simulink model "model_2"  (R2023b)
settings: Solver=FixedStepAuto  StartTime=0.0  StopTime=10  FixedStep=0.001  RelTol=1e-3
undefined symbols (not defined in the file or in its folder): G_d, T, xi_0
settings Model: Creator=Denis  LastModifiedBy=Denis

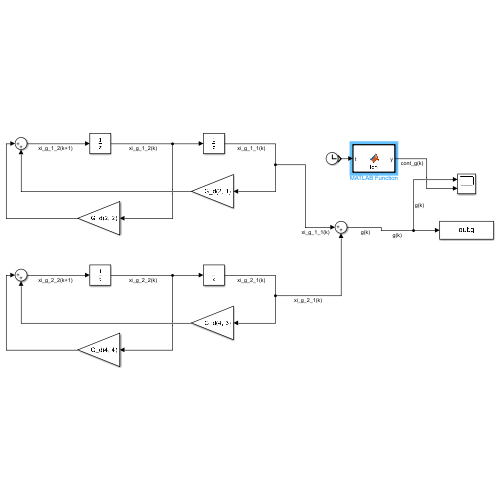
[thumbnail: Simulink's stored preview of the top-level diagram]
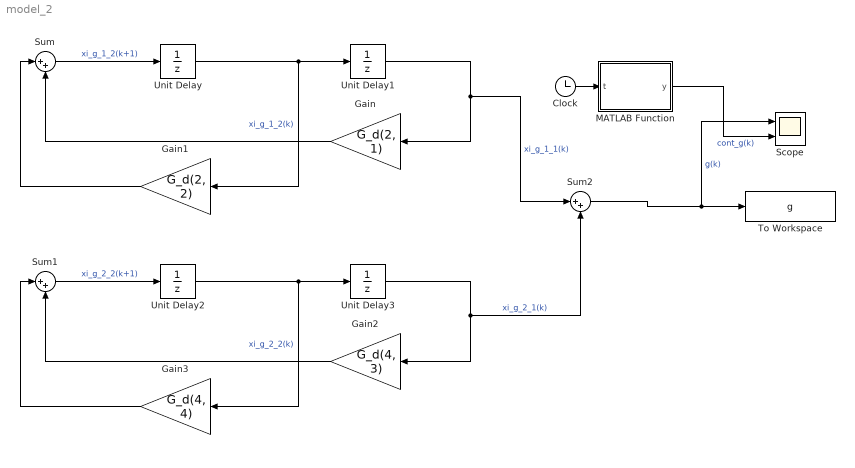
== system model_2 ==
  Clock : Clock
  Gain : Gain  Gain=G_d(2, 1)
  Gain1 : Gain  Gain=G_d(2, 2)
  Gain2 : Gain  Gain=G_d(4, 3)
  Gain3 : Gain  Gain=G_d(4, 4)
  MATLAB Function : MATLAB Function  TreatAsAtomicUnit=on
  Scope : Scope  NumInputPorts=2
  Sum : Sum  Inputs=|++
  Sum1 : Sum  Inputs=|++
  Sum2 : Sum  Inputs=|++
  To Workspace : ToWorkspace  VariableName=g  SaveFormat=Timeseries  SampleTime=-1
  Unit Delay : UnitDelay  InitialCondition=xi_0(2)  SampleTime=T  HasFrameUpgradeWarning=on
  Unit Delay1 : UnitDelay  InitialCondition=xi_0(1)  SampleTime=T  HasFrameUpgradeWarning=on
  Unit Delay2 : UnitDelay  InitialCondition=xi_0(4)  SampleTime=T  HasFrameUpgradeWarning=on
  Unit Delay3 : UnitDelay  InitialCondition=xi_0(3)  SampleTime=T  HasFrameUpgradeWarning=on
  wires:
  Unit Delay1/1 -> Gain/1, Sum2/1  "xi_g_1_1(k)"
  Gain/1 -> Sum/2
  Unit Delay/1 -> Unit Delay1/1, Gain1/1  "xi_g_1_2(k)"
  Gain1/1 -> Sum/1
  Sum/1 -> Unit Delay/1  "xi_g_1_2(k+1)"
  Unit Delay3/1 -> Sum2/2, Gain2/1  "xi_g_2_1(k)"
  Gain2/1 -> Sum1/2
  Unit Delay2/1 -> Unit Delay3/1, Gain3/1  "xi_g_2_2(k)"
  Gain3/1 -> Sum1/1
  Sum1/1 -> Unit Delay2/1  "xi_g_2_2(k+1)"
  Sum2/1 -> Scope/1, To Workspace/1  "g(k)"
  Clock/1 -> MATLAB Function/1(t)
  MATLAB Function/1(y) -> Scope/2  "cont_g(k)"

== matlab function model_2/MATLAB Function ==
  data: t input; y output
function y = fcn(t)
    
y = 2*sin(2*t) + 3*cos(5*t);
end
